simulink model "practica1ejercicio7"  (Simulink 7.5)
settings: Solver=ode45  StartTime=0.0  StopTime=10.0  RelTol=1e-3
settings Model: Creator=Mariano  LastModifiedBy=Mariano

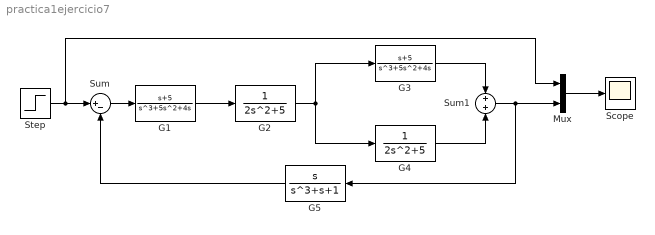
== system practica1ejercicio7 ==
  G1 : TransferFcn  Numerator=[1 5]  Denominator=[1 5 4 0]
  G2 : TransferFcn  Denominator=[2 0 5]
  G3 : TransferFcn  Numerator=[1 5]  Denominator=[1 5 4 0]
  G4 : TransferFcn  Denominator=[2 0 5]
  G5 : TransferFcn  Numerator=[1 0]  Denominator=[1 0 1 1]
  Mux : Mux  Inputs=2
  Scope : Scope
  Step : Step  Time=0  SampleTime=0
  Sum : Sum  Inputs=|+-  OutDataType=fixdt(1, 16)  OutScaling=2^0
  Sum1 : Sum  OutDataType=fixdt(1, 16)  OutScaling=2^0
  wires:
  Step/1 -> Sum/1, Mux/1
  Mux/1 -> Scope/1
  Sum1/1 -> Mux/2, G5/1
  Sum/1 -> G1/1
  G1/1 -> G2/1
  G2/1 -> G3/1, G4/1
  G3/1 -> Sum1/1
  G4/1 -> Sum1/2
  G5/1 -> Sum/2
